simulink model "Project_ACS_Microgrid_Dynamics_Simulation_And_Test_2018a"  (R2018a)
settings: Solver=VariableStepAuto  StartTime=0.0  StopTime=2  MaxStep=1e-4  RelTol=1e-2
undefined symbols (not defined in the file): powergui, rt
libraries: powerlib x25, powerlib_meascontrol x16, simulink x7
(part 1 of 2)
settings Model: Creator=vikasrai89  LastModifiedBy=MdNahidKhan
settings OptimizationCC: LifeSpan=inf
settings DebuggingCC: LibraryContextMissingDiagnostic=warning  SFExecutionAtInitializationDiag=none
settings CodeAppCC: StateflowObjectComments=on

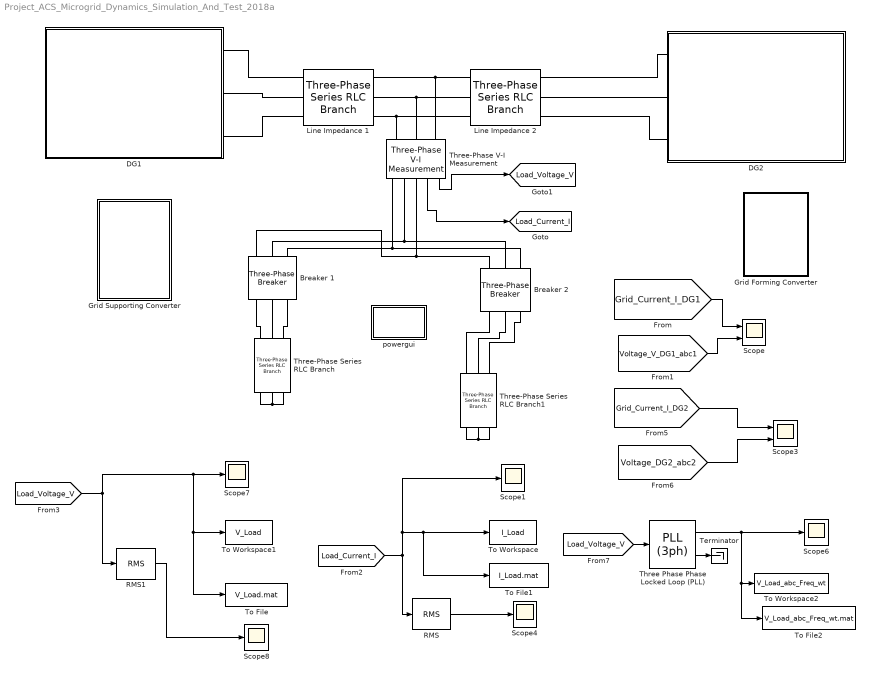
== system Project_ACS_Microgrid_Dynamics_Simulation_And_Test_2018a ==
  Breaker 1 : powerlib/Elements/Three-Phase Breaker  InitialState=closed  SwitchA=on  SwitchB=on  SwitchC=on  SwitchTimes=10/50  External=off  BreakerResistance=0.01  SnubberResistance=1e6  SnubberCapacitance=inf  Measurements=None
      settings: SourceProductName=Simscape Electrical
  Breaker 2 : powerlib/Elements/Three-Phase Breaker  InitialState=open  SwitchA=on  SwitchB=on  SwitchC=on  SwitchTimes=10/50  External=off  BreakerResistance=0.01  SnubberResistance=1e6  SnubberCapacitance=inf  Measurements=None
      settings: SourceProductName=Simscape Electrical
  DG1 : Subsystem  Description=DG!
  DG2 : Subsystem  Description=DG!
  Grid Forming Converter : Subsystem
  Grid Supporting Converter : Subsystem
  Line Impedance 1 : powerlib/Elements/Three-Phase Series RLC Branch  LConnTagsString=A|B|C  RConnTagsString=A|B|C  BranchType=RL  Resistance=1  Inductance=0.01  Capacitance=1e-6  Measurements=None
      settings: SourceProductName=Simscape Electrical
  Line Impedance 2 : powerlib/Elements/Three-Phase Series RLC Branch  LConnTagsString=A|B|C  RConnTagsString=A|B|C  BranchType=RL  Resistance=1  Inductance=0.01  Capacitance=1e-6  Measurements=None
      settings: SourceProductName=Simscape Electrical
  RMS : powerlib_meascontrol/Measurements/RMS  TrueRMS=on  Freq=50  RMSInit=0  Ts=0
      settings: SourceProductName=Simscape Electrical
  RMS1 : powerlib_meascontrol/Measurements/RMS  TrueRMS=on  Freq=50  RMSInit=0  Ts=0
      settings: SourceProductName=Simscape Electrical
  Scope : Scope  NumInputPorts=2
  Scope{1,4,6..8} (5 alike) : Scope
      Scope1 settings: AttributesFormatString=Load Current
      Scope4 settings: AttributesFormatString=RMS Value of Load Current
      Scope6 settings: AttributesFormatString=Change in Frequency
      Scope7 settings: AttributesFormatString=Load Voltage
      Scope8 settings: AttributesFormatString=RMS Value of Load Voltage
  Scope3 : Scope  NumInputPorts=2
  Terminator : Terminator
  Three Phase Phase Locked Loop (PLL) : powerlib_meascontrol/PLL/PLL (3ph)  Fmin=45  Par_Init=[0, 50]  ParK=[180, 3200, 1]  TcD=1e-4  MaxRateChangeFreq=12  FilterCutOffFreq=25  Ts=0  AGC=on
      settings: SourceProductName=Simscape Electrical
  Three-Phase Series RLC Branch : powerlib/Elements/Three-Phase Series RLC Branch  LConnTagsString=A|B|C  RConnTagsString=A|B|C  BranchType=R  Resistance=50  Inductance=1e-3  Capacitance=1e-6  Measurements=None
      settings: AttributesFormatString=Resistive Load 1 = 50 Ω  SourceProductName=Simscape Electrical
  Three-Phase Series RLC Branch1 : powerlib/Elements/Three-Phase Series RLC Branch  LConnTagsString=A|B|C  RConnTagsString=A|B|C  BranchType=R  Resistance=40  Inductance=1e-3  Capacitance=1e-6  Measurements=None
      settings: AttributesFormatString=Resistive Load 2 = 40 Ω  SourceProductName=Simscape Electrical
  Three-Phase V-I Measurement : powerlib/Measurements/Three-Phase V-I Measurement  VoltageMeasurement=phase-to-ground  SetLabelV=off  LabelV=Vabc  Vpu=off  VpuLL=off  CurrentMeasurement=yes  SetLabelI=off  LabelI=Iabc  Ipu=off  Pbase=100e6  Vbase=500e3  OutputType=Complex  PhasorSimulation=off  PSBequivalent=0
      settings: SourceProductName=Simscape Electrical
  To File : ToFile  Filename=V_Load.mat  SaveFormat=Timeseries
  To File1 : ToFile  Filename=I_Load.mat  SaveFormat=Timeseries
  To File2 : ToFile  Filename=V_Load_abc_Freq_wt.mat  SaveFormat=Timeseries
  To Workspace : ToWorkspace  VariableName=I_Load  SaveFormat=Timeseries  SampleTime=-1
  To Workspace1 : ToWorkspace  VariableName=V_Load  SaveFormat=Timeseries  SampleTime=-1
  To Workspace2 : ToWorkspace  VariableName=V_Load_abc_Freq_wt  SaveFormat=Timeseries  SampleTime=-1
  powergui : Subsystem  Priority=1  AncestorBlock=powerlib/powergui  DialogController=POWERSYS.PowerSysDialog  InitFcn=powergui( 'InitFcn_Callback' , gcb , 0 , [ ] );  mask(PSB option menu block){SimulationMode=Continuous, SampleTime=1e-6, frequency=60, Iterations=50, frequencyindice=0, Pbase=100e6, ErrMax=1e-4, UnitsV=kV, UnitsW=MW, buscounter=0, FunctionMessages=off, echomessages=off, EnableUseOfTLC=off, CurrentSourceSwitches=off, DisableSnubberDevices=off, DisableRonSwitches=off, DisableVfSwitches=off, DisplayEquations=off, SolverType=Tustin/Backward Euler (TBE), Interpol=off, ExternalGateDelay=off, methode=off, Ts=100, x0status=blocks, SPID=on, SwTol=0, HookPort=off, RestoreLinks=warning, ResistiveCurrentMeasurement=off, Frange=[0:2:500], Ylog=off, Xlog=on, ShowGrid=off, save=off, variable=ZData, structure=0, ZoomFFT=off, StartTime=0.0, cycles=1, DisplayStyle=1, fundamental=60, FreqAxis=off, MaxFrequency=1000, frequencyindicesteady=1, RmsSteady=1, display=off}
      mask prompts: SimulationMode "Simulation type:"; SampleTime "Sample time (s):"; frequency "Frequency (Hz):"; Iterations "Max iterations"; frequencyindice "Frequency (Hz)"; Pbase "Base power (VA)"; ErrMax "PQ tolerance (pu)"; UnitsV "Voltage units"; UnitsW "Power units"; buscounter "Load flow bus counter"; FunctionMessages "Disable Specialized Power Systems warnings"; echomessages "Display Specialized Power Systems compilation messages"; EnableUseOfTLC "Use TLC file when in Accelerator Simulation Mode and for code generation"; CurrentSourceSwitches "Disable ideal switching"; DisableSnubberDevices "Disable snubbers in switching devices"; DisableRonSwitches "Disable Ron resistances in switching devices"; DisableVfSwitches "Disable forward voltages in switching devices"; DisplayEquations "Display circuit differential equations"; SolverType "Discrete solver"; Interpol "Interpolate switching events"; ExternalGateDelay "Use time-stamped gate signals"; methode "Store switching topologies"; Ts "Buffer size (MBytes):"; x0status "Start simulation with initial electrical states from:"; SPID "Use ideal switching devices"; SwTol "Switch tolerance"; HookPort "Allow multiple powergui blocks"; RestoreLinks "Restore disabled links of Simscape Power Systems ST blocks:"; ResistiveCurrentMeasurement "Use non ideal current measurement blocks (1e-4Ohm internal resistance)"; Frange "Frequency Range"; Ylog "Log impedance"; Xlog "log Frequency"; ShowGrid "grid"; save "Save Data To Workspace"; variable "Variable Name"; structure "Structure Name (PSBFFTSCOPE)"; ZoomFFT "ZoomFFT (PSBFFTSCOPE)"; StartTime "Start Time (PSBFFTSCOPE)"; cycles "Cycles (PSBFFTSCOPE)"; DisplayStyle "Display style (PSBFFTSCOPE)"; fundamental "Fundamental (PSBFFTSCOPE)"; FreqAxis "Frequency Axis (PSBFFTSCOPE)"; MaxFrequency "Max Frequency (PSBFFTSCOPE)"; frequencyindicesteady "Frequency indice (STEADYSTATE)"; RmsSteady "RMS display (STEADYSTATE)"; display "Display Results"
      mask help: Set simulation type, simulation parameters, and preferences.
      mask init:
      | dispMessage = powergui('MaskInitialization',gcb,SimulationMode,SampleTime);
      settings: PreSaveFcn=powergui( 'PreSaveFcn_Callback' , gcb , [ ] , [ ] );  OpenFcn=sps_rtmsupport('OpenFcn',gcbh)
      mask Help: helpview(psbhelp)
      mask TypeOptions SimulationMode: Continuous | Discrete | Phasor
      mask Callback SimulationMode: powergui('SimulationType',[],[],gcb);
      mask TypeOptions UnitsV: V | kV
      mask TypeOptions UnitsW: W | kW | MW
      mask Callback CurrentSourceSwitches: powergui('SimulationType',[],[],gcb);
      mask TypeOptions SolverType: Tustin/Backward Euler (TBE) | Tustin | Backward Euler
      mask Callback SolverType: powergui('SimulationType',[],[],gcb);
      mask Callback Interpol: powergui('SimulationType',[],[],gcb);
      mask Callback ExternalGateDelay: powergui('SimulationType',[],[],gcb);
      mask Callback methode: powergui('SimulationType',[],[],gcb);
      mask TypeOptions x0status: blocks | steady | zero
      mask TypeOptions RestoreLinks: yes | warning | no
      mask Callback display: sps_rtmsupport('parametereditingmodes',gcbh) % Will be executed last in parameter callbacks to ensure mask enable consistency
      mask DialogControl SolverTab Prompt: Solver
      mask DialogControl AutoSolverNote Prompt: To enable the Powergui solver settings, unselect auto (Automatic solver selection) solver in the Simulink solver options.
      mask DialogControl AnalysisTools Prompt: Tools
      mask DialogControl SteadyState Prompt: Steady-State
      mask DialogControl SteadyState Callback: close_system(gcb); power_steadystate(bdroot(gcb),gcb);
      mask DialogControl InitialState Prompt: Initial State
      mask DialogControl InitialState Callback: close_system(gcb); power_initstates(bdroot(gcb),gcb)
      mask DialogControl MachineInitialization Prompt: Machine Initialization
      mask DialogControl MachineInitialization Callback: close_system(gcb); power_loadflow(bdroot(gcb),gcb);
      mask DialogControl ImpedanceMeasurement Prompt: Impedance Measurement
      mask DialogControl ImpedanceMeasurement Callback: close_system(gcb); power_zmeter(bdroot(gcb),gcb);
      mask DialogControl FFTAnalysis Prompt: FFT Analysis
      mask DialogControl FFTAnalysis Callback: close_system(gcb); power_fftscope(bdroot(gcb),gcb);
      mask DialogControl LinearSystemAnalyzer Prompt: Use Linear System Analyzer
      mask DialogControl LinearSystemAnalyzer Callback: close_system(gcb); power_ltiview(bdroot(gcb),gcb);
      mask DialogControl HysteresisDesign Prompt: Hysteresis Design
      mask DialogControl HysteresisDesign Callback: close_system(gcb); power_hysteresis(bdroot(gcb),gcb);
      mask DialogControl RLCLineParameters Prompt: RLC Line Parameters
      mask DialogControl RLCLineParameters Callback: close_system(gcb); power_lineparam(bdroot(gcb),gcb);
      mask DialogControl GenerateReprot Prompt: Generate Report
      mask DialogControl GenerateReprot Callback: close_system(gcb); power_report(bdroot(gcb),gcb);
      mask DialogControl Control14 Prompt: Customize SPS blocks
      mask DialogControl Control14 Callback: close_system(gcb); power_customize;
      mask DialogControl LoadFlow Prompt: Load Flow
      mask DialogControl LoadFlow Callback: close_system(gcb); power_loadflow('-v2',bdroot(gcb));
      mask DialogControl Container14 Prompt: Load flow settings
      mask DialogControl ParameterTabVar012 Prompt: Preferences
      mask Display: color('blue'),disp(dispMessage)
  tag scope: Load_Current_I=global, Load_Voltage_V=global
  wires:
  [Grid_Current_I_DG1] -> Scope/1
  [Voltage_V_DG1_abc1] -> Scope/2
  Three-Phase V-I Measurement/2 -> [Load_Current_I]
  Three-Phase V-I Measurement/1 -> [Load_Voltage_V]
  [Load_Current_I] -> Scope1/1, To File1/1, To Workspace/1, RMS/1
  [Voltage_DG2_abc2] -> Scope3/2
  [Grid_Current_I_DG2] -> Scope3/1
  RMS/1 -> Scope4/1
  RMS1/1 -> Scope8/1
  [Load_Voltage_V] -> Three Phase Phase Locked Loop (PLL)/1
  Three Phase Phase Locked Loop (PLL)/1 -> To File2/1, To Workspace2/1, Scope6/1
  Three Phase Phase Locked Loop (PLL)/2 -> Terminator/1
  [Load_Voltage_V] -> RMS1/1, To File/1, To Workspace1/1, Scope7/1
  connections:
  Line Impedance 2/LConn1 -- Three-Phase V-I Measurement/LConn1 -- Line Impedance 1/RConn1
  Line Impedance 2/LConn2 -- Three-Phase V-I Measurement/LConn2 -- Line Impedance 1/RConn2
  Line Impedance 2/LConn3 -- Three-Phase V-I Measurement/LConn3 -- Line Impedance 1/RConn3
  DG1/RConn1 -- Line Impedance 1/LConn1
  Line Impedance 1/LConn2 -- DG1/RConn2
  DG1/RConn3 -- Line Impedance 1/LConn3
  DG2/RConn1 -- Line Impedance 2/RConn1
  DG2/RConn3 -- Line Impedance 2/RConn3
  Three-Phase Series RLC Branch/LConn2 -- Three-Phase Series RLC Branch/LConn3 -- Three-Phase Series RLC Branch/LConn1
  Breaker 1/RConn1 -- Breaker 2/RConn1 -- Three-Phase V-I Measurement/RConn1
  Breaker 1/RConn2 -- Breaker 2/RConn2 -- Three-Phase V-I Measurement/RConn2
  Three-Phase V-I Measurement/RConn3 -- Breaker 1/RConn3 -- Breaker 2/RConn3
  Three-Phase Series RLC Branch1/LConn3 -- Three-Phase Series RLC Branch1/LConn1 -- Three-Phase Series RLC Branch1/LConn2
  Breaker 1/LConn2 -- Three-Phase Series RLC Branch/RConn2
  Breaker 2/LConn2 -- Three-Phase Series RLC Branch1/RConn2
  Breaker 1/LConn3 -- Three-Phase Series RLC Branch/RConn3
  Breaker 1/LConn1 -- Three-Phase Series RLC Branch/RConn1
  Breaker 2/LConn1 -- Three-Phase Series RLC Branch1/RConn1
  Breaker 2/LConn3 -- Three-Phase Series RLC Branch1/RConn3
  DG2/RConn2 -- Line Impedance 2/RConn2

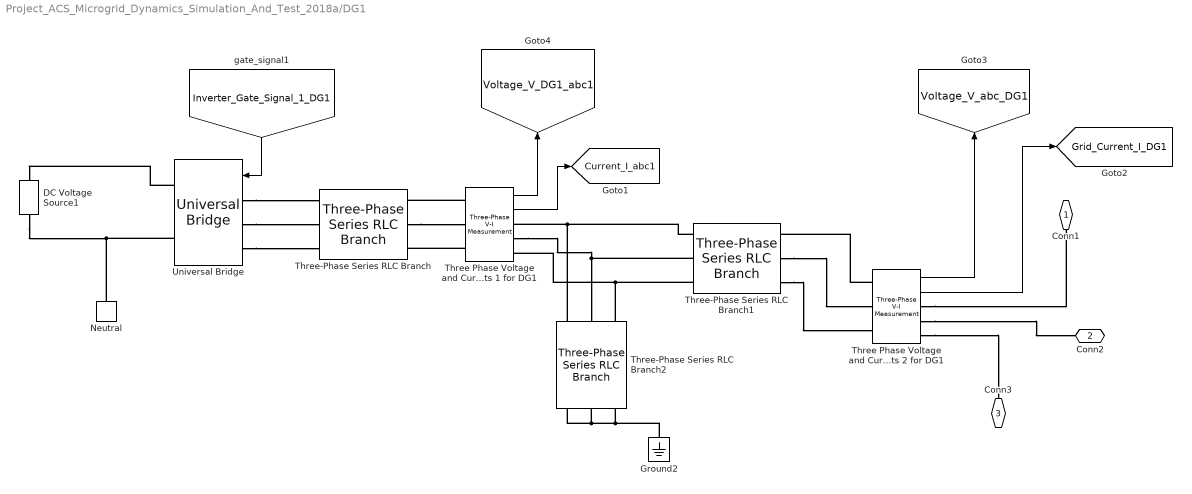
== system Project_ACS_Microgrid_Dynamics_Simulation_And_Test_2018a/DG1 ==
  DC Voltage Source1 : powerlib/Electrical Sources/DC Voltage Source  Amplitude=750  Measurements=Voltage
      settings: SourceProductName=Simscape Electrical
  Ground2 : powerlib/Elements/Ground  LConnTagsString=a
      settings: SourceProductName=Simscape Electrical
  Neutral : powerlib/Elements/Neutral  LConnTagsString=a  NodeNumber=10
      settings: SourceProductName=Simscape Electrical  SourceProductBaseCode=PS
  Three Phase Voltage and Current Measurements 1 for DG1 : powerlib/Measurements/Three-Phase V-I Measurement  VoltageMeasurement=phase-to-ground  SetLabelV=off  LabelV=Vabc  Vpu=off  VpuLL=off  CurrentMeasurement=yes  SetLabelI=off  LabelI=Iabc  Ipu=off  Pbase=100e6  Vbase=500e3  OutputType=Complex  PhasorSimulation=off  PSBequivalent=0
      settings: SourceProductName=Simscape Electrical
  Three Phase Voltage and Current Measurements 2 for DG1 : powerlib/Measurements/Three-Phase V-I Measurement  VoltageMeasurement=phase-to-ground  SetLabelV=off  LabelV=Vabc  Vpu=off  VpuLL=off  CurrentMeasurement=yes  SetLabelI=off  LabelI=Iabc  Ipu=off  Pbase=100e6  Vbase=500e3  OutputType=Complex  PhasorSimulation=off  PSBequivalent=0
      settings: SourceProductName=Simscape Electrical
  Three-Phase Series RLC Branch : powerlib/Elements/Three-Phase Series RLC Branch  LConnTagsString=A|B|C  RConnTagsString=A|B|C  BranchType=L  Resistance=rt  Inductance=0.003  Capacitance=1e-6  Measurements=None
      settings: SourceProductName=Simscape Electrical
  Three-Phase Series RLC Branch1 : powerlib/Elements/Three-Phase Series RLC Branch  LConnTagsString=A|B|C  RConnTagsString=A|B|C  BranchType=L  Resistance=rt  Inductance=0.0015  Capacitance=1e-6  Measurements=None
      settings: SourceProductName=Simscape Electrical
  Three-Phase Series RLC Branch2 : powerlib/Elements/Three-Phase Series RLC Branch  LConnTagsString=A|B|C  RConnTagsString=A|B|C  BranchType=C  Resistance=rt  Inductance=0.003  Capacitance=10e-6  Measurements=Branch voltages and currents
      settings: SourceProductName=Simscape Electrical
  Universal Bridge : powerlib/Power Electronics/Universal Bridge  Arms=3  SnubberResistance=1e5  SnubberCapacitance=inf  Device=IGBT / Diodes  Ron=1e-3  Lon=0  ForwardVoltages="[  0  0  ]"  ForwardVoltage=0  GTOparameters=[ 10e-6 , 20e-6 ]  IGBTparameters=[ 1e-6 , 2e-6 ]  Measurements=None  Measurements_2=None  converterType=Rectifier
      settings: SourceProductName=Simscape Electrical
  Conn1 : PMIOPort  Side=Right
  Conn2 : PMIOPort  Port=2  Side=Right
  Conn3 : PMIOPort  Port=3  Side=Right
  tag scope: Current_I_abc1=global, Grid_Current_I_DG1=global, Voltage_V_DG1_abc1=global, Voltage_V_abc_DG1=global
  wires:
  Three Phase Voltage and Current Measurements 1 for DG1/2 -> [Current_I_abc1]
  [Inverter_Gate_Signal_1_DG1] -> Universal Bridge/1
  Three Phase Voltage and Current Measurements 2 for DG1/1 -> [Voltage_V_abc_DG1]
  Three Phase Voltage and Current Measurements 2 for DG1/2 -> [Grid_Current_I_DG1]
  Three Phase Voltage and Current Measurements 1 for DG1/1 -> [Voltage_V_DG1_abc1]
  connections:
  DC Voltage Source1/LConn1 -- Universal Bridge/RConn2 -- Neutral/LConn1
  Universal Bridge/LConn3 -- Three-Phase Series RLC Branch/LConn3
  Universal Bridge/LConn2 -- Three-Phase Series RLC Branch/LConn2
  Three Phase Voltage and Current Measurements 1 for DG1/LConn3 -- Three-Phase Series RLC Branch/RConn3
  Universal Bridge/LConn1 -- Three-Phase Series RLC Branch/LConn1
  Three Phase Voltage and Current Measurements 1 for DG1/LConn1 -- Three-Phase Series RLC Branch/RConn1
  Three-Phase Series RLC Branch/RConn2 -- Three Phase Voltage and Current Measurements 1 for DG1/LConn2
  Three-Phase Series RLC Branch2/LConn3 -- Three Phase Voltage and Current Measurements 1 for DG1/RConn3 -- Three-Phase Series RLC Branch1/LConn3
  Three-Phase Series RLC Branch2/LConn1 -- Three-Phase Series RLC Branch1/LConn1 -- Three Phase Voltage and Current Measurements 1 for DG1/RConn1
  Three-Phase Series RLC Branch1/LConn2 -- Three Phase Voltage and Current Measurements 1 for DG1/RConn2 -- Three-Phase Series RLC Branch2/LConn2
  Ground2/LConn1 -- Three-Phase Series RLC Branch2/RConn1 -- Three-Phase Series RLC Branch2/RConn2 -- Three-Phase Series RLC Branch2/RConn3
  Universal Bridge/RConn1 -- DC Voltage Source1/RConn1
  Three Phase Voltage and Current Measurements 2 for DG1/RConn2 -- Conn2/RConn1
  Three Phase Voltage and Current Measurements 2 for DG1/RConn1 -- Conn1/RConn1
  Three Phase Voltage and Current Measurements 2 for DG1/RConn3 -- Conn3/RConn1
  Three Phase Voltage and Current Measurements 2 for DG1/LConn1 -- Three-Phase Series RLC Branch1/RConn1
  Three-Phase Series RLC Branch1/RConn2 -- Three Phase Voltage and Current Measurements 2 for DG1/LConn2
  Three-Phase Series RLC Branch1/RConn3 -- Three Phase Voltage and Current Measurements 2 for DG1/LConn3

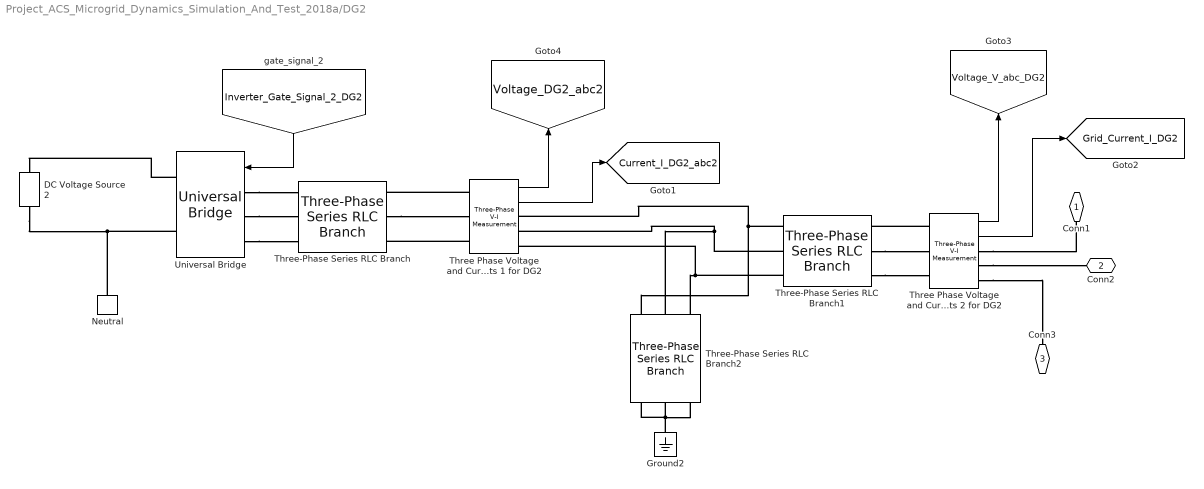
== system Project_ACS_Microgrid_Dynamics_Simulation_And_Test_2018a/DG2 ==
  DC Voltage Source 2 : powerlib/Electrical Sources/DC Voltage Source  Amplitude=750  Measurements=Voltage
      settings: SourceProductName=Simscape Electrical
  Ground2 : powerlib/Elements/Ground  LConnTagsString=a
      settings: SourceProductName=Simscape Electrical
  Neutral : powerlib/Elements/Neutral  LConnTagsString=a  NodeNumber=10
      settings: SourceProductName=Simscape Electrical  SourceProductBaseCode=PS
  Three Phase Voltage and Current Measurements 1 for DG2 : powerlib/Measurements/Three-Phase V-I Measurement  VoltageMeasurement=phase-to-ground  SetLabelV=off  LabelV=Vabc  Vpu=off  VpuLL=off  CurrentMeasurement=yes  SetLabelI=off  LabelI=Iabc  Ipu=off  Pbase=100e6  Vbase=500e3  OutputType=Complex  PhasorSimulation=off  PSBequivalent=0
      settings: SourceProductName=Simscape Electrical
  Three Phase Voltage and Current Measurements 2 for DG2 : powerlib/Measurements/Three-Phase V-I Measurement  VoltageMeasurement=phase-to-ground  SetLabelV=off  LabelV=Vabc  Vpu=off  VpuLL=off  CurrentMeasurement=yes  SetLabelI=off  LabelI=Iabc  Ipu=off  Pbase=100e6  Vbase=500e3  OutputType=Complex  PhasorSimulation=off  PSBequivalent=0
      settings: SourceProductName=Simscape Electrical
  Three-Phase Series RLC Branch : powerlib/Elements/Three-Phase Series RLC Branch  LConnTagsString=A|B|C  RConnTagsString=A|B|C  BranchType=L  Resistance=rt  Inductance=0.003  Capacitance=1e-6  Measurements=None
      settings: SourceProductName=Simscape Electrical
  Three-Phase Series RLC Branch1 : powerlib/Elements/Three-Phase Series RLC Branch  LConnTagsString=A|B|C  RConnTagsString=A|B|C  BranchType=L  Resistance=rt  Inductance=0.0015  Capacitance=1e-6  Measurements=None
      settings: SourceProductName=Simscape Electrical
  Three-Phase Series RLC Branch2 : powerlib/Elements/Three-Phase Series RLC Branch  LConnTagsString=A|B|C  RConnTagsString=A|B|C  BranchType=C  Resistance=rt  Inductance=0.003  Capacitance=10e-6  Measurements=Branch voltages and currents
      settings: SourceProductName=Simscape Electrical
  Universal Bridge : powerlib/Power Electronics/Universal Bridge  Arms=3  SnubberResistance=1e5  SnubberCapacitance=inf  Device=IGBT / Diodes  Ron=1e-3  Lon=0  ForwardVoltages="[  0  0  ]"  ForwardVoltage=0  GTOparameters=[ 10e-6 , 20e-6 ]  IGBTparameters=[ 1e-6 , 2e-6 ]  Measurements=None  Measurements_2=None  converterType=Rectifier
      settings: SourceProductName=Simscape Electrical
  Conn1 : PMIOPort  Side=Right
  Conn2 : PMIOPort  Port=2  Side=Right
  Conn3 : PMIOPort  Port=3  Side=Right
  tag scope: Current_I_DG2_abc2=global, Grid_Current_I_DG2=global, Voltage_DG2_abc2=global, Voltage_V_abc_DG2=global
  wires:
  Three Phase Voltage and Current Measurements 1 for DG2/2 -> [Current_I_DG2_abc2]
  [Inverter_Gate_Signal_2_DG2] -> Universal Bridge/1
  Three Phase Voltage and Current Measurements 2 for DG2/1 -> [Voltage_V_abc_DG2]
  Three Phase Voltage and Current Measurements 2 for DG2/2 -> [Grid_Current_I_DG2]
  Three Phase Voltage and Current Measurements 1 for DG2/1 -> [Voltage_DG2_abc2]
  connections:
  DC Voltage Source 2/LConn1 -- Universal Bridge/RConn2 -- Neutral/LConn1
  Universal Bridge/LConn3 -- Three-Phase Series RLC Branch/LConn3
  Universal Bridge/LConn2 -- Three-Phase Series RLC Branch/LConn2
  Three Phase Voltage and Current Measurements 1 for DG2/LConn3 -- Three-Phase Series RLC Branch/RConn3
  Universal Bridge/LConn1 -- Three-Phase Series RLC Branch/LConn1
  Three Phase Voltage and Current Measurements 1 for DG2/LConn1 -- Three-Phase Series RLC Branch/RConn1
  Three-Phase Series RLC Branch/RConn2 -- Three Phase Voltage and Current Measurements 1 for DG2/LConn2
  Three-Phase Series RLC Branch2/LConn3 -- Three-Phase Series RLC Branch1/LConn3 -- Three Phase Voltage and Current Measurements 1 for DG2/RConn3
  Three-Phase Series RLC Branch2/LConn1 -- Three Phase Voltage and Current Measurements 1 for DG2/RConn1 -- Three-Phase Series RLC Branch1/LConn1
  Three-Phase Series RLC Branch2/LConn2 -- Three Phase Voltage and Current Measurements 1 for DG2/RConn2 -- Three-Phase Series RLC Branch1/LConn2
  Ground2/LConn1 -- Three-Phase Series RLC Branch2/RConn3 -- Three-Phase Series RLC Branch2/RConn1 -- Three-Phase Series RLC Branch2/RConn2
  Universal Bridge/RConn1 -- DC Voltage Source 2/RConn1
  Three Phase Voltage and Current Measurements 2 for DG2/RConn2 -- Conn2/RConn1
  Three Phase Voltage and Current Measurements 2 for DG2/RConn1 -- Conn1/RConn1
  Three Phase Voltage and Current Measurements 2 for DG2/RConn3 -- Conn3/RConn1
  Three Phase Voltage and Current Measurements 2 for DG2/LConn1 -- Three-Phase Series RLC Branch1/RConn1
  Three-Phase Series RLC Branch1/RConn2 -- Three Phase Voltage and Current Measurements 2 for DG2/LConn2
  Three-Phase Series RLC Branch1/RConn3 -- Three Phase Voltage and Current Measurements 2 for DG2/LConn3

== system Project_ACS_Microgrid_Dynamics_Simulation_And_Test_2018a/Grid Forming Converter ==
  Current Control Loop2 : Subsystem
  Voltage Control Loop2 : Subsystem
  w* : Constant  Value=2*pi*50
  wires:
  Voltage Control Loop2/1(Id*) -> Current Control Loop2/1(Id*)
  Voltage Control Loop2/2(Iq*) -> Current Control Loop2/2(Iq*)
  w*/1 -> Voltage Control Loop2/1(w*)

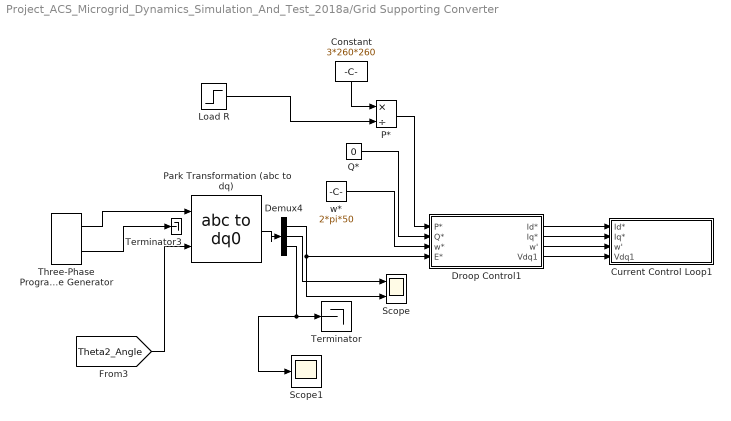
== system Project_ACS_Microgrid_Dynamics_Simulation_And_Test_2018a/Grid Supporting Converter ==
  Constant : Constant  Value=3*260*260
  Current Control Loop1 : Subsystem
  Demux4 : Demux  Outputs=3
  Droop Control1 : Subsystem
  Load R : Step  Time=0.2  Before=50  After=40  SampleTime=0
  P* : Product  Inputs=*/
  Park Transformation (abc to dq) : powerlib_meascontrol/Transformations/abc to dq0  Alignment=90 degrees behind phase A axis
      settings: SourceProductName=Simscape Electrical
  Q* : Constant  Value=0
  Scope : Scope  NumInputPorts=2
  Scope1 : Scope
  Terminator : Terminator
  Terminator3 : Terminator
  Three-Phase Programmable Generator : powerlib_meascontrol/Pulse & Signal Generators/Three-Phase Programmable Generator  Par_Vps=[450, 0, 50]  VariationEntity=None  VariationType=Ramp  VariationStep=-0.5  VariationRate=10  VariationMag=0.3  VariationFreq=2  Par_Timing_Variation="[0.2  1.2]"  SinglePhase=on  Yampli=[1 0.2 1.2 1.0]  Xtime=[0 0.1 0.15 0.2]  HarmonicGeneration=off  Par_HarmoA="[3  5  -25 0]"  Par_HarmoB="[5  10  35  2]"  Par_Timing_Harmo="[ 0.05  99]"  Ts=0
      settings: SourceProductName=Simscape Electrical  SourceProductBaseCode=PS
  w* : Constant  Value=2*pi*50
  wires:
  Demux4/1 -> Scope/2, Droop Control1/4(E*)
  Constant/1 -> P*/1
  w*/1 -> Droop Control1/3(w*)
  P*/1 -> Droop Control1/1(P*)
  Load R/1 -> P*/2
  Q*/1 -> Droop Control1/2(Q*)
  Droop Control1/2(Iq*) -> Current Control Loop1/2(Iq*)
  Droop Control1/1(Id*) -> Current Control Loop1/1(Id*)
  Droop Control1/3(w') -> Current Control Loop1/3(w')
  Droop Control1/4(Vdq1) -> Current Control Loop1/4(Vdq1)
  Three-Phase Programmable Generator/1 -> Park Transformation (abc to dq)/1
  [Theta2_Angle] -> Park Transformation (abc to dq)/2
  Park Transformation (abc to dq)/1 -> Demux4/1
  Demux4/3 -> Scope1/1, Terminator/1
  Demux4/2 -> Scope/1
  Three-Phase Programmable Generator/2 -> Terminator3/1

== system Project_ACS_Microgrid_Dynamics_Simulation_And_Test_2018a/powergui ==
  note: Graphical user interface for the analysis of
      | Simscape Power Systems (Specialized Technology) circuits.
      | Place the Powergui block in the top-level of your model and double-click
      | on it to open the GUI.
  EquivalentModel1 : Subsystem  mask{SwTol=SwTol}
      mask prompts: SwTol "SwitchTolerance"
      mask init:
      | S  = GetDataForEquivalentModel('SPID',gcbh,SwTol);
      mask Display:
      | color('blue')
      | disp('EQUIVALENT CIRCUIT\nSPID')
  Ground : Ground
  Terminator : Terminator
  wires:
  Ground/1 -> Terminator/1

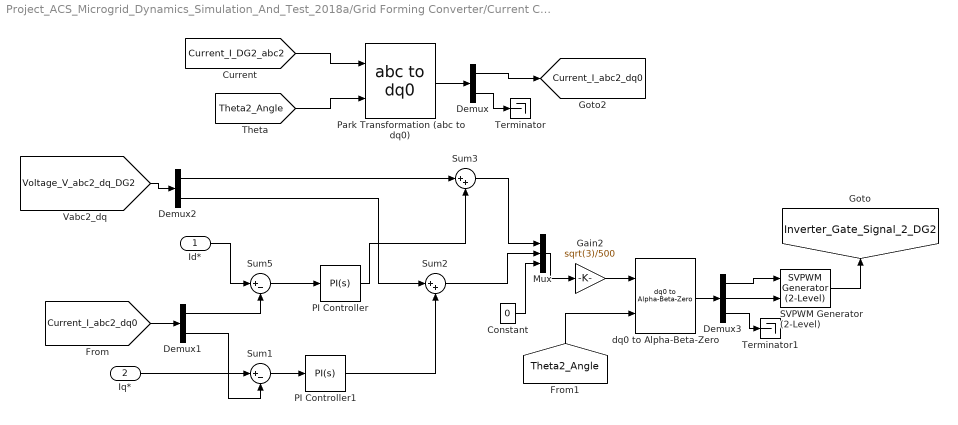
== system Project_ACS_Microgrid_Dynamics_Simulation_And_Test_2018a/Grid Forming Converter/Current Control Loop2 ==
  Id* : Inport
  Iq* : Inport  Port=2
  Constant : Constant  Value=0
  Demux : Demux  Outputs=[2;1]
  Demux1 : Demux  Outputs=2
  Demux2 : Demux  Outputs=2
  Demux3 : Demux  Outputs=3
  Gain2 : Gain  Gain=sqrt(3)/500
  Mux : Mux  Inputs=3
  PI Controller : simulink/Continuous/PID Controller  Controller=PI  Form=Parallel  TimeDomain=Continuous-time  SampleTime=-1  IntegratorMethod=Forward Euler  FilterMethod=Forward Euler  ControllerParametersSource=internal  P=18.84  I=11843.52  D=0  UseFilter=on  N=100  TunerSelectOption=Transfer Function Based (PID Tuner App)  InitialConditionSource=internal  InitialConditionForIntegrator=0  InitialConditionForFilter=0  DifferentiatorICPrevScaledInput=0  ExternalReset=none  TrackingMode=off  Kt=1  LimitOutput=off  UpperSaturationLimit=inf  LowerSaturationLimit=-inf  LinearizeAsGain=on  AntiWindupMode=none  Kb=1  POutMin=[]  POutMax=[]  IOutMin=[]  IOutMax=[]  DOutMin=[]  DOutMax=[]  NOutMin=[]  NOutMax=[]  SumOutMin=[]  SumOutMax=[]  SaturationOutMin=[]  SaturationOutMax=[]  PParamMin=[]  PParamMax=[]  IParamMin=[]  IParamMax=[]  DParamMin=[]  DParamMax=[]  NParamMin=[]  NParamMax=[]  KbParamMin=[]  KbParamMax=[]  KtParamMin=[]  KtParamMax=[]  KbOutMin=[]  KbOutMax=[]  KtOutMin=[]  KtOutMax=[]  IntegratorOutMin=[]  IntegratorOutMax=[]  FilterOutMin=[]  FilterOutMax=[]  SumI1OutMin=[]  SumI1OutMax=[]  SumI2OutMin=[]  SumI2OutMax=[]  SumI3OutMin=[]  SumI3OutMax=[]  SumDOutMin=[]  SumDOutMax=[]  DifferentiatorOutMin=[]  DifferentiatorOutMax=[]  FilterDiffOutCoefMin=[]  FilterDiffOutCoefMax=[]  ReciprocalOutMin=[]  ReciprocalOutMax=[]  SumDenOutMin=[]  SumDenOutMax=[]  SumNumOutMin=[]  SumNumOutMax=[]  DivideOutMin=[]  DivideOutMax=[]  IntegratorContinuousStateAttributes=''  IntegratorStateMustResolveToSignalObject=off  IntegratorRTWStateStorageClass=Auto  FilterContinuousStateAttributes=''  FilterStateMustResolveToSignalObject=off  FilterRTWStateStorageClass=Auto
  PI Controller1 : simulink/Continuous/PID Controller  Controller=PI  Form=Parallel  TimeDomain=Continuous-time  SampleTime=-1  IntegratorMethod=Forward Euler  FilterMethod=Forward Euler  ControllerParametersSource=internal  P=18.84  I=11843.52  D=0  UseFilter=on  N=100  TunerSelectOption=Transfer Function Based (PID Tuner App)  InitialConditionSource=internal  InitialConditionForIntegrator=0  InitialConditionForFilter=0  DifferentiatorICPrevScaledInput=0  ExternalReset=none  TrackingMode=off  Kt=1  LimitOutput=off  UpperSaturationLimit=inf  LowerSaturationLimit=-inf  LinearizeAsGain=on  AntiWindupMode=none  Kb=1  POutMin=[]  POutMax=[]  IOutMin=[]  IOutMax=[]  DOutMin=[]  DOutMax=[]  NOutMin=[]  NOutMax=[]  SumOutMin=[]  SumOutMax=[]  SaturationOutMin=[]  SaturationOutMax=[]  PParamMin=[]  PParamMax=[]  IParamMin=[]  IParamMax=[]  DParamMin=[]  DParamMax=[]  NParamMin=[]  NParamMax=[]  KbParamMin=[]  KbParamMax=[]  KtParamMin=[]  KtParamMax=[]  KbOutMin=[]  KbOutMax=[]  KtOutMin=[]  KtOutMax=[]  IntegratorOutMin=[]  IntegratorOutMax=[]  FilterOutMin=[]  FilterOutMax=[]  SumI1OutMin=[]  SumI1OutMax=[]  SumI2OutMin=[]  SumI2OutMax=[]  SumI3OutMin=[]  SumI3OutMax=[]  SumDOutMin=[]  SumDOutMax=[]  DifferentiatorOutMin=[]  DifferentiatorOutMax=[]  FilterDiffOutCoefMin=[]  FilterDiffOutCoefMax=[]  ReciprocalOutMin=[]  ReciprocalOutMax=[]  SumDenOutMin=[]  SumDenOutMax=[]  SumNumOutMin=[]  SumNumOutMax=[]  DivideOutMin=[]  DivideOutMax=[]  IntegratorContinuousStateAttributes=''  IntegratorStateMustResolveToSignalObject=off  IntegratorRTWStateStorageClass=Auto  FilterContinuousStateAttributes=''  FilterStateMustResolveToSignalObject=off  FilterRTWStateStorageClass=Auto
  Park Transformation (abc to dq0) : powerlib_meascontrol/Transformations/abc to dq0  Alignment=90 degrees behind phase A axis
      settings: SourceProductName=Simscape Electrical
  SVPWM Generator (2-Level) : powerlib_meascontrol/Pulse & Signal Generators/SVPWM Generator (2-Level)  InputType=alpha-beta components  SwitchingPattern=Pattern #1  Fc=10000  ParUref=[1 0 50]  Ts=0
      settings: SourceProductName=Simscape Electrical  SourceProductBaseCode=PS
  Sum1 : Sum  Inputs=|+-
  Sum2 : Sum  Inputs=|++
  Sum3 : Sum  Inputs=|++
  Sum5 : Sum  Inputs=|+-
  Terminator : Terminator
  Terminator1 : Terminator
  dq0 to Alpha-Beta-Zero : powerlib_meascontrol/Transformations/dq0 to Alpha-Beta-Zero  Alignment=90 degrees behind phase A axis
      settings: SourceProductName=Simscape Electrical  SourceProductBaseCode=PS
  tag scope: Current_I_abc2_dq0=global, Inverter_Gate_Signal_2_DG2=global
  wires:
  Demux/2 -> Terminator/1
  [Current_I_DG2_abc2] -> Park Transformation (abc to dq0)/1
  Park Transformation (abc to dq0)/1 -> Demux/1
  Sum5/1 -> PI Controller/1
  Sum3/1 -> Mux/1
  Constant/1 -> Mux/3
  Sum2/1 -> Mux/2
  [Theta2_Angle] -> Park Transformation (abc to dq0)/2
  Id*/1 -> Sum5/1
  [Current_I_abc2_dq0] -> Demux1/1
  Demux1/1 -> Sum5/2
  Iq*/1 -> Sum1/1
  Demux1/2 -> Sum1/2
  Sum1/1 -> PI Controller1/1
  Demux2/1 -> Sum3/1
  [Voltage_V_abc2_dq_DG2] -> Demux2/1
  PI Controller/1 -> Sum3/2
  PI Controller1/1 -> Sum2/2
  Demux2/2 -> Sum2/1
  Demux3/2 -> SVPWM Generator (2-Level)/2
  [Theta2_Angle] -> dq0 to Alpha-Beta-Zero/2
  dq0 to Alpha-Beta-Zero/1 -> Demux3/1
  Demux3/3 -> Terminator1/1
  Demux3/1 -> SVPWM Generator (2-Level)/1
  SVPWM Generator (2-Level)/1 -> [Inverter_Gate_Signal_2_DG2]
  Gain2/1 -> dq0 to Alpha-Beta-Zero/1
  Mux/1 -> Gain2/1
  Demux/1 -> [Current_I_abc2_dq0]

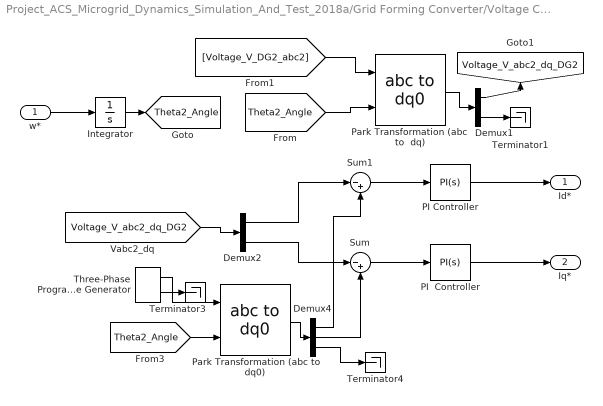
== system Project_ACS_Microgrid_Dynamics_Simulation_And_Test_2018a/Grid Forming Converter/Voltage Control Loop2 ==
  w* : Inport
  Demux1 : Demux  Outputs=[2;1]
  Demux2 : Demux  Outputs=2
  Demux4 : Demux  Outputs=3
  Integrator : Integrator
  PI  Controller : simulink/Continuous/PID Controller  Controller=PI  Form=Parallel  TimeDomain=Continuous-time  SampleTime=-1  IntegratorMethod=Forward Euler  FilterMethod=Forward Euler  ControllerParametersSource=internal  P=0.0628  I=39.45  D=0  UseFilter=on  N=100  TunerSelectOption=Transfer Function Based (PID Tuner App)  InitialConditionSource=internal  InitialConditionForIntegrator=0  InitialConditionForFilter=0  DifferentiatorICPrevScaledInput=0  ExternalReset=none  TrackingMode=off  Kt=1  LimitOutput=off  UpperSaturationLimit=inf  LowerSaturationLimit=-inf  LinearizeAsGain=on  AntiWindupMode=none  Kb=1  POutMin=[]  POutMax=[]  IOutMin=[]  IOutMax=[]  DOutMin=[]  DOutMax=[]  NOutMin=[]  NOutMax=[]  SumOutMin=[]  SumOutMax=[]  SaturationOutMin=[]  SaturationOutMax=[]  PParamMin=[]  PParamMax=[]  IParamMin=[]  IParamMax=[]  DParamMin=[]  DParamMax=[]  NParamMin=[]  NParamMax=[]  KbParamMin=[]  KbParamMax=[]  KtParamMin=[]  KtParamMax=[]  KbOutMin=[]  KbOutMax=[]  KtOutMin=[]  KtOutMax=[]  IntegratorOutMin=[]  IntegratorOutMax=[]  FilterOutMin=[]  FilterOutMax=[]  SumI1OutMin=[]  SumI1OutMax=[]  SumI2OutMin=[]  SumI2OutMax=[]  SumI3OutMin=[]  SumI3OutMax=[]  SumDOutMin=[]  SumDOutMax=[]  DifferentiatorOutMin=[]  DifferentiatorOutMax=[]  FilterDiffOutCoefMin=[]  FilterDiffOutCoefMax=[]  ReciprocalOutMin=[]  ReciprocalOutMax=[]  SumDenOutMin=[]  SumDenOutMax=[]  SumNumOutMin=[]  SumNumOutMax=[]  DivideOutMin=[]  DivideOutMax=[]  IntegratorContinuousStateAttributes=''  IntegratorStateMustResolveToSignalObject=off  IntegratorRTWStateStorageClass=Auto  FilterContinuousStateAttributes=''  FilterStateMustResolveToSignalObject=off  FilterRTWStateStorageClass=Auto
  PI Controller : simulink/Continuous/PID Controller  Controller=PI  Form=Parallel  TimeDomain=Continuous-time  SampleTime=-1  IntegratorMethod=Forward Euler  FilterMethod=Forward Euler  ControllerParametersSource=internal  P=0.0628  I=39.45  D=0  UseFilter=on  N=100  TunerSelectOption=Transfer Function Based (PID Tuner App)  InitialConditionSource=internal  InitialConditionForIntegrator=0  InitialConditionForFilter=0  DifferentiatorICPrevScaledInput=0  ExternalReset=none  TrackingMode=off  Kt=1  LimitOutput=off  UpperSaturationLimit=inf  LowerSaturationLimit=-inf  LinearizeAsGain=on  AntiWindupMode=none  Kb=1  POutMin=[]  POutMax=[]  IOutMin=[]  IOutMax=[]  DOutMin=[]  DOutMax=[]  NOutMin=[]  NOutMax=[]  SumOutMin=[]  SumOutMax=[]  SaturationOutMin=[]  SaturationOutMax=[]  PParamMin=[]  PParamMax=[]  IParamMin=[]  IParamMax=[]  DParamMin=[]  DParamMax=[]  NParamMin=[]  NParamMax=[]  KbParamMin=[]  KbParamMax=[]  KtParamMin=[]  KtParamMax=[]  KbOutMin=[]  KbOutMax=[]  KtOutMin=[]  KtOutMax=[]  IntegratorOutMin=[]  IntegratorOutMax=[]  FilterOutMin=[]  FilterOutMax=[]  SumI1OutMin=[]  SumI1OutMax=[]  SumI2OutMin=[]  SumI2OutMax=[]  SumI3OutMin=[]  SumI3OutMax=[]  SumDOutMin=[]  SumDOutMax=[]  DifferentiatorOutMin=[]  DifferentiatorOutMax=[]  FilterDiffOutCoefMin=[]  FilterDiffOutCoefMax=[]  ReciprocalOutMin=[]  ReciprocalOutMax=[]  SumDenOutMin=[]  SumDenOutMax=[]  SumNumOutMin=[]  SumNumOutMax=[]  DivideOutMin=[]  DivideOutMax=[]  IntegratorContinuousStateAttributes=''  IntegratorStateMustResolveToSignalObject=off  IntegratorRTWStateStorageClass=Auto  FilterContinuousStateAttributes=''  FilterStateMustResolveToSignalObject=off  FilterRTWStateStorageClass=Auto
  Park Transformation (abc  to  dq) : powerlib_meascontrol/Transformations/abc to dq0  Alignment=90 degrees behind phase A axis
      settings: SourceProductName=Simscape Electrical
  Park Transformation (abc to dq0) : powerlib_meascontrol/Transformations/abc to dq0  Alignment=90 degrees behind phase A axis
      settings: SourceProductName=Simscape Electrical
  Sum : Sum  Inputs=|-+
  Sum1 : Sum  Inputs=|-+
  Terminator1 : Terminator
  Terminator3 : Terminator
  Terminator4 : Terminator
  Three-Phase Programmable Generator : powerlib_meascontrol/Pulse & Signal Generators/Three-Phase Programmable Generator  Par_Vps=[450, 0, 50]  VariationEntity=None  VariationType=Ramp  VariationStep=-0.5  VariationRate=10  VariationMag=0.3  VariationFreq=2  Par_Timing_Variation="[0.2  1.2]"  SinglePhase=on  Yampli=[1 0.2 1.2 1.0]  Xtime=[0 0.1 0.15 0.2]  HarmonicGeneration=off  Par_HarmoA="[3  5  -25 0]"  Par_HarmoB="[5  10  35  2]"  Par_Timing_Harmo="[ 0.05  99]"  Ts=0
      settings: SourceProductName=Simscape Electrical  SourceProductBaseCode=PS
  Id* : Outport
  Iq* : Outport  Port=2
  tag scope: Theta2_Angle=global, Voltage_V_abc2_dq_DG2=global
  wires:
  Park Transformation (abc  to  dq)/1 -> Demux1/1
  Demux1/1 -> [Voltage_V_abc2_dq_DG2]
  [Voltage_V_DG2_abc2] -> Park Transformation (abc  to  dq)/1
  Demux1/2 -> Terminator1/1
  [Theta2_Angle] -> Park Transformation (abc  to  dq)/2
  [Voltage_V_abc2_dq_DG2] -> Demux2/1
  Demux2/2 -> Sum/1
  Sum1/1 -> PI Controller/1
  Sum/1 -> PI  Controller/1
  PI Controller/1 -> Id*/1
  PI  Controller/1 -> Iq*/1
  Park Transformation (abc to dq0)/1 -> Demux4/1
  [Theta2_Angle] -> Park Transformation (abc to dq0)/2
  Three-Phase Programmable Generator/1 -> Park Transformation (abc to dq0)/1
  Three-Phase Programmable Generator/2 -> Terminator3/1
  Demux4/2 -> Sum/2
  Demux4/3 -> Terminator4/1
  w*/1 -> Integrator/1
  Integrator/1 -> [Theta2_Angle]
  Demux4/1 -> Sum1/2
  Demux2/1 -> Sum1/1

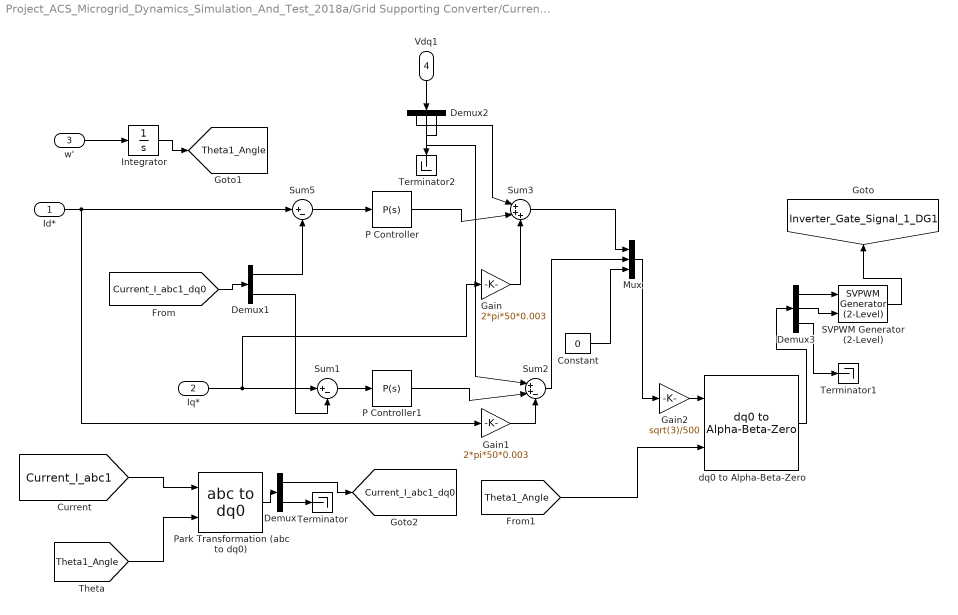
== system Project_ACS_Microgrid_Dynamics_Simulation_And_Test_2018a/Grid Supporting Converter/Current Control Loop1 ==
  Id* : Inport
  Iq* : Inport  Port=2
  w' : Inport  Port=3
  Vdq1 : Inport  Port=4
  Constant : Constant  Value=0
  Demux : Demux  Outputs=[2;1]
  Demux1 : Demux  Outputs=2
  Demux2 : Demux  Outputs=3
  Demux3 : Demux  Outputs=3
  Gain : Gain  Gain=2*pi*50*0.003
  Gain1 : Gain  Gain=2*pi*50*0.003
  Gain2 : Gain  Gain=sqrt(3)/500
  Integrator : Integrator
  Mux : Mux  Inputs=3
  P Controller : simulink/Continuous/PID Controller  Controller=P  Form=Parallel  TimeDomain=Continuous-time  SampleTime=-1  IntegratorMethod=Forward Euler  FilterMethod=Forward Euler  ControllerParametersSource=internal  P=18.84  I=11843.52  D=0  UseFilter=on  N=100  TunerSelectOption=Transfer Function Based (PID Tuner App)  InitialConditionSource=internal  InitialConditionForIntegrator=0  InitialConditionForFilter=0  DifferentiatorICPrevScaledInput=0  ExternalReset=none  TrackingMode=off  Kt=1  LimitOutput=off  UpperSaturationLimit=inf  LowerSaturationLimit=-inf  LinearizeAsGain=on  AntiWindupMode=none  Kb=1  POutMin=[]  POutMax=[]  IOutMin=[]  IOutMax=[]  DOutMin=[]  DOutMax=[]  NOutMin=[]  NOutMax=[]  SumOutMin=[]  SumOutMax=[]  SaturationOutMin=[]  SaturationOutMax=[]  PParamMin=[]  PParamMax=[]  IParamMin=[]  IParamMax=[]  DParamMin=[]  DParamMax=[]  NParamMin=[]  NParamMax=[]  KbParamMin=[]  KbParamMax=[]  KtParamMin=[]  KtParamMax=[]  KbOutMin=[]  KbOutMax=[]  KtOutMin=[]  KtOutMax=[]  IntegratorOutMin=[]  IntegratorOutMax=[]  FilterOutMin=[]  FilterOutMax=[]  SumI1OutMin=[]  SumI1OutMax=[]  SumI2OutMin=[]  SumI2OutMax=[]  SumI3OutMin=[]  SumI3OutMax=[]  SumDOutMin=[]  SumDOutMax=[]  DifferentiatorOutMin=[]  DifferentiatorOutMax=[]  FilterDiffOutCoefMin=[]  FilterDiffOutCoefMax=[]  ReciprocalOutMin=[]  ReciprocalOutMax=[]  SumDenOutMin=[]  SumDenOutMax=[]  SumNumOutMin=[]  SumNumOutMax=[]  DivideOutMin=[]  DivideOutMax=[]  IntegratorContinuousStateAttributes=''  IntegratorStateMustResolveToSignalObject=off  IntegratorRTWStateStorageClass=Auto  FilterContinuousStateAttributes=''  FilterStateMustResolveToSignalObject=off  FilterRTWStateStorageClass=Auto
  P Controller1 : simulink/Continuous/PID Controller  Controller=P  Form=Parallel  TimeDomain=Continuous-time  SampleTime=-1  IntegratorMethod=Forward Euler  FilterMethod=Forward Euler  ControllerParametersSource=internal  P=18.84  I=11843.52  D=0  UseFilter=on  N=100  TunerSelectOption=Transfer Function Based (PID Tuner App)  InitialConditionSource=internal  InitialConditionForIntegrator=0  InitialConditionForFilter=0  DifferentiatorICPrevScaledInput=0  ExternalReset=none  TrackingMode=off  Kt=1  LimitOutput=off  UpperSaturationLimit=inf  LowerSaturationLimit=-inf  LinearizeAsGain=on  AntiWindupMode=none  Kb=1  POutMin=[]  POutMax=[]  IOutMin=[]  IOutMax=[]  DOutMin=[]  DOutMax=[]  NOutMin=[]  NOutMax=[]  SumOutMin=[]  SumOutMax=[]  SaturationOutMin=[]  SaturationOutMax=[]  PParamMin=[]  PParamMax=[]  IParamMin=[]  IParamMax=[]  DParamMin=[]  DParamMax=[]  NParamMin=[]  NParamMax=[]  KbParamMin=[]  KbParamMax=[]  KtParamMin=[]  KtParamMax=[]  KbOutMin=[]  KbOutMax=[]  KtOutMin=[]  KtOutMax=[]  IntegratorOutMin=[]  IntegratorOutMax=[]  FilterOutMin=[]  FilterOutMax=[]  SumI1OutMin=[]  SumI1OutMax=[]  SumI2OutMin=[]  SumI2OutMax=[]  SumI3OutMin=[]  SumI3OutMax=[]  SumDOutMin=[]  SumDOutMax=[]  DifferentiatorOutMin=[]  DifferentiatorOutMax=[]  FilterDiffOutCoefMin=[]  FilterDiffOutCoefMax=[]  ReciprocalOutMin=[]  ReciprocalOutMax=[]  SumDenOutMin=[]  SumDenOutMax=[]  SumNumOutMin=[]  SumNumOutMax=[]  DivideOutMin=[]  DivideOutMax=[]  IntegratorContinuousStateAttributes=''  IntegratorStateMustResolveToSignalObject=off  IntegratorRTWStateStorageClass=Auto  FilterContinuousStateAttributes=''  FilterStateMustResolveToSignalObject=off  FilterRTWStateStorageClass=Auto
  Park Transformation (abc to dq0) : powerlib_meascontrol/Transformations/abc to dq0  Alignment=90 degrees behind phase A axis
      settings: SourceProductName=Simscape Electrical
  SVPWM Generator (2-Level) : powerlib_meascontrol/Pulse & Signal Generators/SVPWM Generator (2-Level)  InputType=alpha-beta components  SwitchingPattern=Pattern #1  Fc=10000  ParUref=[1 0 50]  Ts=0
      settings: SourceProductName=Simscape Electrical  SourceProductBaseCode=PS
  Sum1 : Sum  Inputs=|+-
  Sum2 : Sum  Inputs=|++-
  Sum3 : Sum  Inputs=|+++
  Sum5 : Sum  Inputs=|+-
  Terminator : Terminator
  Terminator1 : Terminator
  Terminator2 : Terminator
  dq0 to Alpha-Beta-Zero : powerlib_meascontrol/Transformations/dq0 to Alpha-Beta-Zero  Alignment=90 degrees behind phase A axis
      settings: SourceProductName=Simscape Electrical  SourceProductBaseCode=PS
  tag scope: Current_I_abc1_dq0=global, Inverter_Gate_Signal_1_DG1=global, Theta1_Angle=global
  wires:
  Demux/2 -> Terminator/1
  [Current_I_abc1] -> Park Transformation (abc to dq0)/1
  Demux/1 -> [Current_I_abc1_dq0]
  Park Transformation (abc to dq0)/1 -> Demux/1
  Sum5/1 -> P Controller/1
  Sum3/1 -> Mux/1
  Gain/1 -> Sum3/3
  Constant/1 -> Mux/3
  Sum2/1 -> Mux/2
  [Theta1_Angle] -> Park Transformation (abc to dq0)/2
  Id*/1 -> Sum5/1, Gain1/1
  [Current_I_abc1_dq0] -> Demux1/1
  Demux1/1 -> Sum5/2
  Iq*/1 -> Gain/1, Sum1/1
  Demux1/2 -> Sum1/2
  Sum1/1 -> P Controller1/1
  Demux2/1 -> Sum3/1
  P Controller/1 -> Sum3/2
  Gain1/1 -> Sum2/3
  P Controller1/1 -> Sum2/2
  Demux2/2 -> Sum2/1
  [Theta1_Angle] -> dq0 to Alpha-Beta-Zero/2
  Mux/1 -> Gain2/1
  Gain2/1 -> dq0 to Alpha-Beta-Zero/1
  w'/1 -> Integrator/1
  Integrator/1 -> [Theta1_Angle]
  Vdq1/1 -> Demux2/1
  Demux2/3 -> Terminator2/1
  Demux3/3 -> Terminator1/1
  Demux3/1 -> SVPWM Generator (2-Level)/1
  Demux3/2 -> SVPWM Generator (2-Level)/2
  dq0 to Alpha-Beta-Zero/1 -> Demux3/1
  SVPWM Generator (2-Level)/1 -> [Inverter_Gate_Signal_1_DG1]

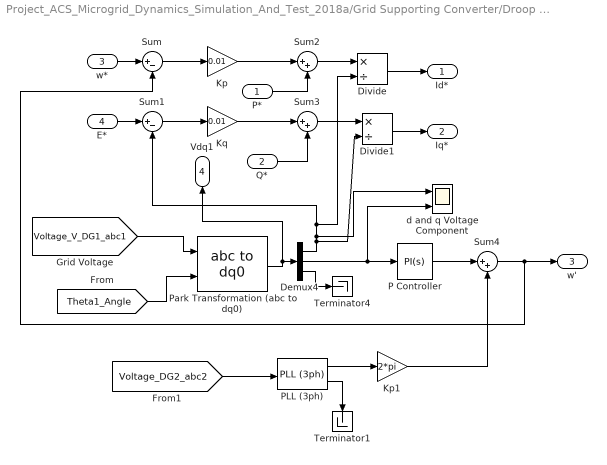
== system Project_ACS_Microgrid_Dynamics_Simulation_And_Test_2018a/Grid Supporting Converter/Droop Control1 ==
  P* : Inport
  Q* : Inport  Port=2
  w* : Inport  Port=3
  E* : Inport  Port=4
  Demux4 : Demux  Outputs=3
  Divide : Product  Inputs=*/
  Divide1 : Product  Inputs=*/
  Kp : Gain  Gain=0.01
  Kp1 : Gain  Gain=2*pi
  Kq : Gain  Gain=0.01
  P Controller : simulink/Continuous/PID Controller  Controller=PI  Form=Parallel  TimeDomain=Continuous-time  SampleTime=-1  IntegratorMethod=Forward Euler  FilterMethod=Forward Euler  ControllerParametersSource=internal  P=30  I=100  D=0  UseFilter=on  N=100  TunerSelectOption=Transfer Function Based (PID Tuner App)  InitialConditionSource=internal  InitialConditionForIntegrator=0  InitialConditionForFilter=0  DifferentiatorICPrevScaledInput=0  ExternalReset=none  TrackingMode=off  Kt=1  LimitOutput=off  UpperSaturationLimit=inf  LowerSaturationLimit=-inf  LinearizeAsGain=on  AntiWindupMode=none  Kb=1  POutMin=[]  POutMax=[]  IOutMin=[]  IOutMax=[]  DOutMin=[]  DOutMax=[]  NOutMin=[]  NOutMax=[]  SumOutMin=[]  SumOutMax=[]  SaturationOutMin=[]  SaturationOutMax=[]  PParamMin=[]  PParamMax=[]  IParamMin=[]  IParamMax=[]  DParamMin=[]  DParamMax=[]  NParamMin=[]  NParamMax=[]  KbParamMin=[]  KbParamMax=[]  KtParamMin=[]  KtParamMax=[]  KbOutMin=[]  KbOutMax=[]  KtOutMin=[]  KtOutMax=[]  IntegratorOutMin=[]  IntegratorOutMax=[]  FilterOutMin=[]  FilterOutMax=[]  SumI1OutMin=[]  SumI1OutMax=[]  SumI2OutMin=[]  SumI2OutMax=[]  SumI3OutMin=[]  SumI3OutMax=[]  SumDOutMin=[]  SumDOutMax=[]  DifferentiatorOutMin=[]  DifferentiatorOutMax=[]  FilterDiffOutCoefMin=[]  FilterDiffOutCoefMax=[]  ReciprocalOutMin=[]  ReciprocalOutMax=[]  SumDenOutMin=[]  SumDenOutMax=[]  SumNumOutMin=[]  SumNumOutMax=[]  DivideOutMin=[]  DivideOutMax=[]  IntegratorContinuousStateAttributes=''  IntegratorStateMustResolveToSignalObject=off  IntegratorRTWStateStorageClass=Auto  FilterContinuousStateAttributes=''  FilterStateMustResolveToSignalObject=off  FilterRTWStateStorageClass=Auto
  PLL (3ph) : powerlib_meascontrol/PLL/PLL (3ph)  Fmin=45  Par_Init=[0, 50]  ParK=[180, 3200, 1]  TcD=1e-4  MaxRateChangeFreq=12  FilterCutOffFreq=25  Ts=0  AGC=on
      settings: SourceProductName=Simscape Electrical
  Park Transformation (abc to dq0) : powerlib_meascontrol/Transformations/abc to dq0  Alignment=90 degrees behind phase A axis
      settings: SourceProductName=Simscape Electrical
  Sum : Sum  Inputs=|+-
  Sum1 : Sum  Inputs=|+-
  Sum2 : Sum  Inputs=|++
  Sum3 : Sum  Inputs=|++
  Sum4 : Sum  Inputs=|++
  Terminator1 : Terminator
  Terminator4 : Terminator
  d and q Voltage Component : Scope  NumInputPorts=2
  Id* : Outport
  Iq* : Outport  Port=2
  w' : Outport  Port=3
  Vdq1 : Outport  Port=4
  wires:
  Sum/1 -> Kp/1
  Sum1/1 -> Kq/1
  Kp/1 -> Sum2/1
  Kq/1 -> Sum3/1
  Sum2/1 -> Divide/1
  [Theta1_Angle] -> Park Transformation (abc to dq0)/2
  Demux4/3 -> Terminator4/1
  Park Transformation (abc to dq0)/1 -> Vdq1/1, Demux4/1
  P*/1 -> Sum2/2
  Q*/1 -> Sum3/2
  w*/1 -> Sum/1
  E*/1 -> Sum1/1
  Divide/1 -> Id*/1
  Divide1/1 -> Iq*/1
  Sum3/1 -> Divide1/1
  P Controller/1 -> Sum4/1
  Sum4/1 -> w'/1, Sum/2
  Demux4/2 -> d and q Voltage Component/2, P Controller/1
  Demux4/1 -> Divide1/2, d and q Voltage Component/1, Divide/2, Sum1/2
  Kp1/1 -> Sum4/2
  [Voltage_DG2_abc2] -> PLL (3ph)/1
  PLL (3ph)/1 -> Kp1/1
  PLL (3ph)/2 -> Terminator1/1
  [Voltage_V_DG1_abc1] -> Park Transformation (abc to dq0)/1

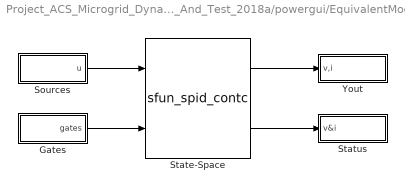
== system Project_ACS_Microgrid_Dynamics_Simulation_And_Test_2018a/powergui/EquivalentModel1 ==
  Gates : Subsystem
  Sources : Subsystem
  State-Space : S-Function  FunctionName=sfun_spid_contc  Parameters=S.Mg, [S.nb.x S.nb.u S.nb.y S.nb.s], S.x0, S.MgColNames, S.SwitchVf, S.SwitchType, S.SwitchGateInitialValue, S.SwitchTolerance,S.SaveMatrices,S.BufferSize  SFunctionDeploymentMode=off  EnableBusSupport=off
  Status : Subsystem
  Yout : Subsystem
  wires:
  State-Space/1 -> Yout/1(v,i)
  State-Space/2 -> Status/1(v&i)
  Gates/1(gates) -> State-Space/2
  Sources/1(u) -> State-Space/1

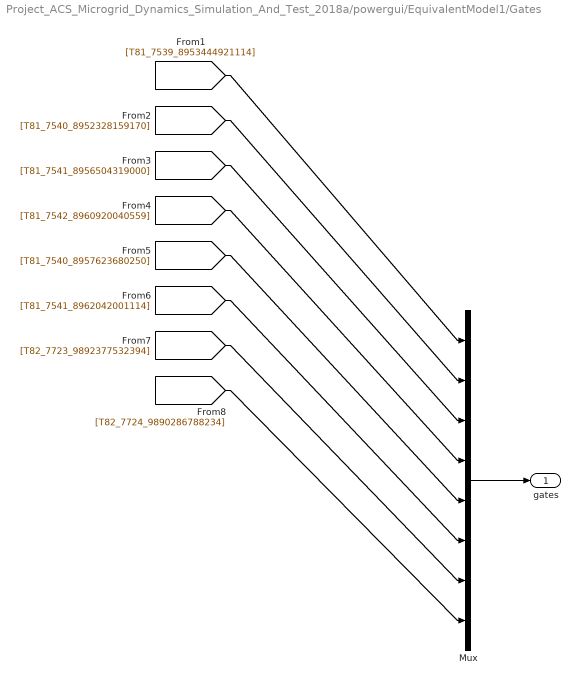
== system Project_ACS_Microgrid_Dynamics_Simulation_And_Test_2018a/powergui/EquivalentModel1/Gates ==
  Mux : Mux  Inputs=[1 1 1 1 1 1 6 6]
  gates : Outport
  wires:
  Mux/1 -> gates/1
  [T81_7539_8953444921114] -> Mux/1
  [T81_7540_8952328159170] -> Mux/2
  [T81_7541_8956504319000] -> Mux/3
  [T81_7542_8960920040559] -> Mux/4
  [T81_7540_8957623680250] -> Mux/5
  [T81_7541_8962042001114] -> Mux/6
  [T82_7723_9892377532394] -> Mux/7
  [T82_7724_9890286788234] -> Mux/8

== system Project_ACS_Microgrid_Dynamics_Simulation_And_Test_2018a/powergui/EquivalentModel1/Sources ==
  Mux : Mux  Inputs=[1 1]
  u : Outport
  wires:
  Mux/1 -> u/1
  [T84_7744_9878518442886] -> Mux/1
  [T85_7778_9872990660975] -> Mux/2

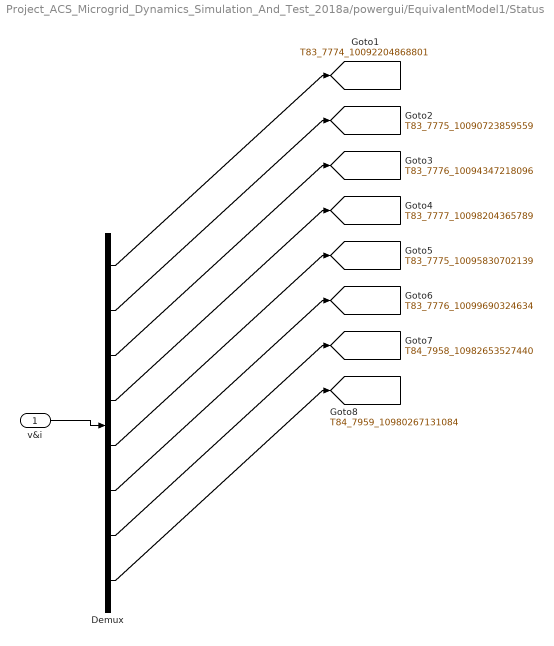
== system Project_ACS_Microgrid_Dynamics_Simulation_And_Test_2018a/powergui/EquivalentModel1/Status ==
  v&i : Inport
  Demux : Demux  Outputs=[2 2 2 2 2 2 12 12]
  tag scope: T83_7774_10092204868801=global, T83_7775_10090723859559=global, T83_7775_10095830702139=global, T83_7776_10094347218096=global, T83_7776_10099690324634=global, T83_7777_10098204365789=global, T84_7958_10982653527440=global, T84_7959_10980267131084=global
  wires:
  v&i/1 -> Demux/1
  Demux/1 -> [T83_7774_10092204868801]
  Demux/2 -> [T83_7775_10090723859559]
  Demux/3 -> [T83_7776_10094347218096]
  Demux/4 -> [T83_7777_10098204365789]
  Demux/5 -> [T83_7775_10095830702139]
  Demux/6 -> [T83_7776_10099690324634]
  Demux/7 -> [T84_7958_10982653527440]
  Demux/8 -> [T84_7959_10980267131084]
